simulink model "OneM"  (R2022b)
settings: Solver=VariableStepAuto  StartTime=0.0  StopTime=30  MaxStep=1e-5  MinStep=1e-6  RelTol=1e-5
settings Model: Creator=yeyi5  LastModifiedBy=yeyi5

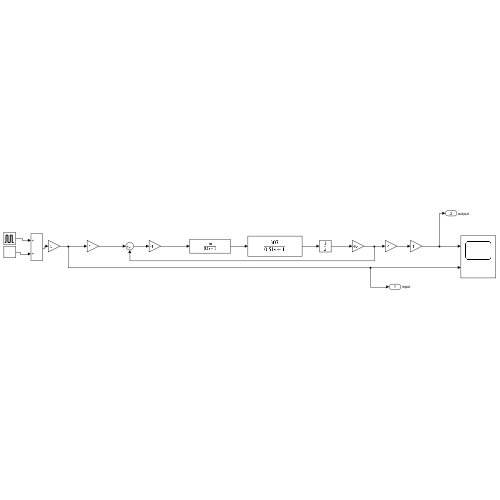
[thumbnail: Simulink's stored preview of the top-level diagram]
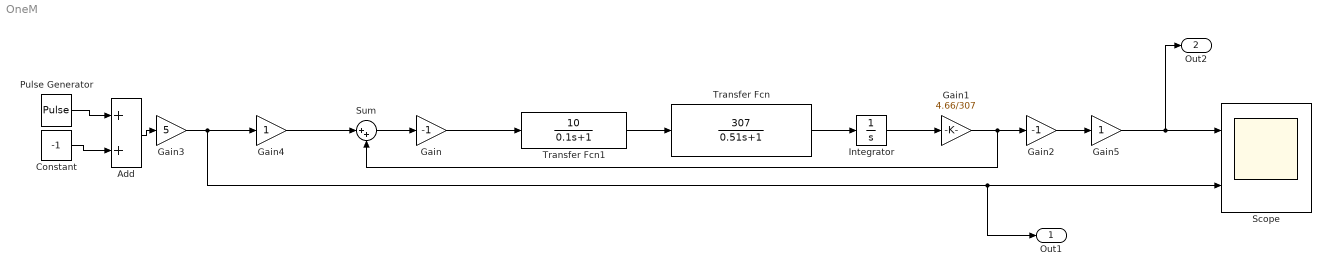
== system OneM ==
  Add : Sum
  Constant : Constant  Value=-1
  Gain : Gain  Gain=-1
  Gain1 : Gain  Gain=4.66/307
  Gain2 : Gain  Gain=-1
  Gain3 : Gain  Gain=5
  Gain4 : Gain
  Gain5 : Gain
  Integrator : Integrator
  Pulse Generator : DiscretePulseGenerator  PulseType=Time based  Amplitude=2  Period=20  PulseWidth=50
  Scope : Scope  NumInputPorts=2
  Sum : Sum  Inputs=|++
  Transfer Fcn : TransferFcn  Numerator=[307]  Denominator=[0.51 1]
  Transfer Fcn1 : TransferFcn  Numerator=[10]  Denominator="[0.1  1]"
  Out1 : Outport  SignalName=input
  Out2 : Outport  Port=2  SignalName=output
  wires:
  Gain1/1 -> Sum/2, Gain2/1
  Gain2/1 -> Gain5/1
  Add/1 -> Gain3/1
  Integrator/1 -> Gain1/1
  Transfer Fcn/1 -> Integrator/1
  Sum/1 -> Gain/1
  Constant/1 -> Add/2
  Pulse Generator/1 -> Add/1
  Transfer Fcn1/1 -> Transfer Fcn/1
  Gain3/1 -> Gain4/1, Out1/1, Scope/2
  Gain/1 -> Transfer Fcn1/1
  Gain4/1 -> Sum/1
  Gain5/1 -> Out2/1, Scope/1
